simulink model "Milestone3_Code_excl4Way"  (R2023a)
settings: Solver=FixedStepDiscrete  StartTime=0.0  StopTime=50  FixedStep=0.01  RelTol=1e-3  EnableMultiTasking=on
undefined symbols (not defined in the file): DiscIntNeverNeededParam
libraries: arduinolib x14, simulink x3, hdlsllib x2, slpidlib x1, mobileRoboticsTrainingLib x1, arduinosensorlib x1
(part 2 of 2)

== stateflow chart Milestone3_Code_excl4Way/Motion Control1/Intersection Navigation1 ==
  note: Basic Description
      | Default: Curve Navigation controls the velocity and angular velocity
      |
      | When infrared sensor 1 or 4 (IR1 and IR4) detect a black line, this Intersection Navigation subsystem takes control and calls the leftTurn or rightTurn procedure respectively.
      | Intersection procedure (same for both leftTurn or rightTurn):
      | 	Increment branchCounter to keep track of the number of branches.
      | 	Move forward a small distance to align with the turn.
      | 	Rotate in the correct direction until the middle two sensors detect a line again.
      | 	Pass control to Curve Navigation to navigate the offshoot.
      | 	If the offshoot comes to an end (all sensors detect white), rotate 180 degrees and navigate back to the main path.
      | 	If the offshoot ends in a detect line (all sensors detect black), stop, send a signal to the Object Detection subsystem to measure for an object, rotate 180 degrees and navigate back to the main path.
      | 		Add branch number from branchCounter to objectMap to indicate this branch has an object.
      | 	Pass control to Curve Navigation to navigate the offshoot returning to the main path.
      | 	When the peripheral sensors detect a black line again (meaning the robot has returned to the intersection with the main branch), control is passed to Intersection Navigation.
      | 	Move forward a small distance to align with the turn.
      | 	Rotate in the correct direction until the middle two sensors detect a line again.
      | 	Pass control back to Curve Navigation to continue traversing the main path.
      |
      | If all sensors detect black whilst the robot is on the main path, the endOfMaze procedure is called.
      | endOfMaze procedure:
      | 	Stop
      | 	Use objectMap to determine how many objects were discovered.
      | 	Find the branch number of the object with the smallest distance, saved to branchWithObject.
      | 		objectCounter provides number of object with smallest distance measured.
      | 		Obtain the n'th number in objectMap to determine the branch number containing said object (where n = objectCounter)
      | 	Invert branchWithObject such that it provides the number of the branch starting from the end of the maze.
      | 	Set renavigating to HIGH.
      |
      | Renavigating Procedure:
      | 	Rotate 180 degrees to re-traverse the maze.
      | 	set branchCounter to 0.
      | 	Pass control to Curve Navigation to renavigate maze.
      | 	If intersection is detected, increment branchCounter.
      | 	If branchCounter is equal to branchWithObject at an intersection, turn into that offshoot.
      | 	Pass control to Curve Navigation to navigate offshoot.
      | 	If all sensors detect black at the "detect object line", come to a stop.
  note: Note to self:
      | Make sure all blocks with forward velocity use curve-following algorithm (never move forward blindly)
      |
      | Neaten up blocks
      |
      | Add 4way navigation
      |
      | Make back and forth smaller (will need to be adjusted for real life speed)
  state analyseIntersection
    state returnToIntersection
      entry: distance0 = distance;
      state FollowTrack
        %middle two sense black
        velocity = -0.05;
        angular_velocity = 0;
      state TurnLeft
        entry:
        velocity = 0;
        angular_velocity = -2;
      state TurnRight
        entry:
        velocity = 0;
        angular_velocity = 2;
      (default) -> analyseIntersection.returnToIntersection.FollowTrack
      analyseIntersection.returnToIntersection.TurnRight -> analyseIntersection.returnToIntersection.FollowTrack : [IR3 == 0 && IR2 == 0]
      analyseIntersection.returnToIntersection.TurnLeft -> analyseIntersection.returnToIntersection.FollowTrack : [IR3 == 0 && IR2 == 0]
      analyseIntersection.returnToIntersection.FollowTrack -> analyseIntersection.returnToIntersection.TurnRight [order 2] : [IR2 == 1]
      analyseIntersection.returnToIntersection.FollowTrack -> analyseIntersection.returnToIntersection.TurnLeft [order 1] : [IR3 == 1]
    state moveForward
      entry: distance0 = distance;
      state FollowTrack
        %middle two sense black
        velocity = 1;
        angular_velocity = 0;
      state TurnRight
        entry:
        velocity = 0;
        angular_velocity = 2;
      state TurnLeft
        entry:
        velocity = 0;
        angular_velocity = -2;
      analyseIntersection.moveForward.TurnLeft -> analyseIntersection.moveForward.FollowTrack : [IR3 == 0 && IR2 == 0]
      analyseIntersection.moveForward.FollowTrack -> analyseIntersection.moveForward.TurnLeft [order 1] : [IR3 == 1]
      analyseIntersection.moveForward.TurnRight -> analyseIntersection.moveForward.FollowTrack : [IR3 == 0 && IR2 == 0]
      analyseIntersection.moveForward.FollowTrack -> analyseIntersection.moveForward.TurnRight [order 2] : [IR2 == 1]
      (default) -> analyseIntersection.moveForward.FollowTrack
    state chooseIntersectionType
      %left turn
      %extreme left turn
      %right turn
      %extreme right turn
      %end of maze
      %4-way junction
      entry: velocity = 0;
      angular_velocity = 0;
    state commenceIntersectionControl
      entry: velocity = 0;
    (default) -> analyseIntersection.moveForward
    chooseIntersectionType -> returnToIntersection [order 2] : [(IR2 == 0 || IR3 == 0)]
    analyseIntersection.moveForward -> chooseIntersectionType : [abs(distance0 - distance) >= 0.3]
    returnToIntersection -> commenceIntersectionControl : [abs(distance0 - distance) >= 0.3]
    (junction 486) -> returnToIntersection : {finishMaze = 1;}
    chooseIntersectionType -> (junction 486) [order 3] : [IR1 + IR2 + IR3 + IR4 == 4]{fourWay = 0;}
    chooseIntersectionType -> (junction 486) [order 1] : [IR1 + IR2 + IR3 + IR4 == 0]{fourWay = 0;}
  note: if fourway doesn't work now:
      | have it pick up if another intersection is ever picked up in the slight move forward, and then limit forward movement massivly.
      | If another interesction in opposite direction was ever picked up - four way
  state endOfMaze
    %procedure to locate position of closest object once maze is completed
    entry: velocity = 0;
    angular_velocity = 0;
    num = objectMap;
    while num > 0
    len = len + 1;
    num = fix(num/10);
    end
    branchWithObject = mod(fix(objectMap/10^(len - objectCounter)), 10);
    branchWithObject = branchCounter - branchWithObject + 1
    exit:
    renavigating = 1;
  state fullRotation
    %rotate 180 degrees to renavigate maze
    entry: phi0 = phi;
    during:
    velocity = 0;
    angular_velocity = -1;
  note: if fullInter == 1:
      | if all black:
  state followMain
    state TurnRight
      entry:
      velocity = 0;
      angular_velocity = 2;
    state FollowTrack
      %middle two sense black
      velocity = 1;
      angular_velocity = 0;
    state TurnLeft
      entry:
      velocity = 0;
      angular_velocity = -2;
    (default) -> followMain.FollowTrack
    followMain.FollowTrack -> followMain.TurnLeft [order 1] : [IR3 == 1]
    followMain.TurnRight -> followMain.FollowTrack : [IR3 == 0 && IR2 == 0]
    followMain.TurnLeft -> followMain.FollowTrack : [IR3 == 0 && IR2 == 0]
    followMain.FollowTrack -> followMain.TurnRight [order 2] : [IR2 == 1]
    (junction 442) -> followMain.FollowTrack
    (junction 440) -> followMain.FollowTrack
  state Wait
  state leftTurn
    %procedure for navigating an offshoot to the right of the main path
    state Rotate
      entry:  branchCounter = branchCounter +1
      state moveForward
        entry: velocity = 1;
      state rotateOffPath
        entry:
        velocity = 0;
        angular_velocity = -1;
      state rotateOntoPath
      (default) -> leftTurn.Rotate.moveForward
      leftTurn.Rotate.moveForward -> leftTurn.Rotate.rotateOffPath : [IR1 == 1]
      leftTurn.Rotate.rotateOffPath -> (junction 365) : [IR2 == 1 && IR3 == 1]
      (junction 365) -> leftTurn.Rotate.rotateOntoPath
    state returnToMain
      state FollowTrack
        %middle two sense black
        velocity = 1;
        angular_velocity = 0;
      state TurnRight
        entry:
        velocity = 0;
        angular_velocity = 2;
      state TurnLeft1
        entry:
        velocity = 0;
        angular_velocity = -2;
      (default) -> leftTurn.returnToMain.FollowTrack
      (junction 469) -> leftTurn.returnToMain.FollowTrack
      (junction 472) -> leftTurn.returnToMain.FollowTrack
      TurnLeft1 -> (junction 469) : [IR3 == 0 && IR2 == 0]
      leftTurn.returnToMain.TurnRight -> (junction 472) : [IR3 == 0 && IR2 == 0]
      leftTurn.returnToMain.FollowTrack -> (junction 471) [order 2] : [IR2 == 1]
      leftTurn.returnToMain.FollowTrack -> (junction 470) [order 1] : [IR3 == 1]
      (junction 471) -> leftTurn.returnToMain.TurnRight
      (junction 470) -> TurnLeft1
    state leftToMain
      state moveForward
        entry: velocity = 1;
      state rotateOntoPath
      state rotateOffPath
        entry:
        velocity = 0;
        angular_velocity = 1;
      (default) -> leftTurn.leftToMain.moveForward
      leftTurn.leftToMain.moveForward -> leftTurn.leftToMain.rotateOffPath : [IR1 == 1]
      (junction 393) -> leftTurn.leftToMain.rotateOntoPath
      leftTurn.leftToMain.rotateOffPath -> (junction 393) : [IR2 == 1 && IR3 == 1]
    state navigateOffshoot
      state FollowTrack
        %middle two sense black
        velocity = 1;
        angular_velocity = 0;
      state TurnLeft
        entry:
        velocity = 0;
        angular_velocity = -2;
      state TurnRight
        entry:
        velocity = 0;
        angular_velocity = 2;
      (default) -> leftTurn.navigateOffshoot.FollowTrack
      leftTurn.navigateOffshoot.FollowTrack -> (junction 460) [order 2] : [IR2 == 1]
      (junction 460) -> leftTurn.navigateOffshoot.TurnRight
      leftTurn.navigateOffshoot.FollowTrack -> (junction 463) [order 1] : [IR3 == 1]
      (junction 463) -> leftTurn.navigateOffshoot.TurnLeft
      (junction 461) -> leftTurn.navigateOffshoot.FollowTrack : [IR3 == 0 && IR2 == 0]
      (junction 462) -> leftTurn.navigateOffshoot.FollowTrack
      leftTurn.navigateOffshoot.TurnRight -> (junction 461)
      leftTurn.navigateOffshoot.TurnLeft -> (junction 462) : [IR3 == 0 && IR2 == 0]
    state fullRotation
      %rotate 180 degrees
      entry: phi0 = phi;
      during:
      velocity = 0;
      angular_velocity = -4;
    state stopAndMeasure
      entry:
      velocity = 0;
      angular_velocity = 0;
      collectMeasurement = 1;
      exit:
      collectMeasurement = 0;
    state finalStop
      velocity = 0;
      angular_velocity = 0;
    (default) -> leftTurn.Rotate
    leftTurn.Rotate.rotateOntoPath -> leftTurn.navigateOffshoot : [IR2 == 0]
    leftTurn.returnToMain -> leftToMain : [IR1 == 0]
    leftTurn.fullRotation -> leftTurn.returnToMain : [abs(phi - phi0) > 2.793 && abs(phi - phi0) < 3.491 && IR2 == 0 && IR3 == 0]
    leftTurn.navigateOffshoot -> (junction 263) [order 2]
    (junction 263) -> (junction 264) : [IR1 + IR2 + IR3 + IR4 == 0 && renavigating == 1]
    leftTurn.navigateOffshoot -> (junction 216) [order 1] : [IR1 == 1 && IR2 == 1 && IR3 == 1 && IR4 == 1]
    (junction 216) -> leftTurn.fullRotation
    leftTurn.navigateOffshoot -> leftTurn.stopAndMeasure [order 3] : [IR1 == 0 && IR2 == 0 && IR3 == 0 && IR4 ==0]{objectMap = objectMap*10 + branchCounter;} %detect or stop line
    leftTurn.stopAndMeasure -> leftTurn.fullRotation : after(1, sec) [measurementComplete == 1]
    (junction 264) -> leftTurn.finalStop
  state rightTurn
    %procedure for navigating an offshoot to the right of the main path
    state returnToMain
      state FollowTrack
        %middle two sense black
        velocity = 1;
        angular_velocity = 0;
      state TurnLeft
        entry:
        velocity = 0;
        angular_velocity = -2;
      state TurnRight
        entry:
        velocity = 0;
        angular_velocity = 2;
      (default) -> rightTurn.returnToMain.FollowTrack
      rightTurn.returnToMain.FollowTrack -> rightTurn.returnToMain.TurnRight [order 2] : [IR2 == 1]
      rightTurn.returnToMain.TurnRight -> rightTurn.returnToMain.FollowTrack : [IR3 == 0 && IR2 == 0]
      rightTurn.returnToMain.FollowTrack -> rightTurn.returnToMain.TurnLeft [order 1] : [IR3 == 1]
      rightTurn.returnToMain.TurnLeft -> rightTurn.returnToMain.FollowTrack : [IR3 == 0 && IR2 == 0]
    state Rotate
      entry:  branchCounter = branchCounter +1
      state moveForward
        entry: velocity = 1;
      state rotateOffPath
        entry:
        velocity = 0;
        angular_velocity = 1;
      state rotateOntoPath
      (default) -> rightTurn.Rotate.moveForward
      rightTurn.Rotate.moveForward -> rightTurn.Rotate.rotateOffPath : [IR4 == 1]
      rightTurn.Rotate.rotateOffPath -> (junction 311) : [IR2 == 1 && IR3 == 1]
      (junction 311) -> rightTurn.Rotate.rotateOntoPath
    state rightToMain
      %turn right back onto the main path
      state moveForward
        entry: velocity = 1;
      state rotateOffPath
        entry:
        velocity = 0;
        angular_velocity = 1;
      state rotateOntoPath
      (default) -> rightTurn.rightToMain.moveForward
      rightTurn.rightToMain.moveForward -> rightTurn.rightToMain.rotateOffPath : [IR4 == 1]
      rightTurn.rightToMain.rotateOffPath -> (junction 357) : [IR2 == 1 && IR3 == 1]
      (junction 357) -> rightTurn.rightToMain.rotateOntoPath
    state navigateOffshoot
      state FollowTrack
        %middle two sense black
        velocity = 1;
        angular_velocity = 0;
      state TurnLeft
        entry:
        velocity = 0;
        angular_velocity = -2;
      state TurnRight1
        entry:
        velocity = 0;
        angular_velocity = 2;
      rightTurn.navigateOffshoot.FollowTrack -> (junction 448) [order 2] : [IR2 == 1]
      rightTurn.navigateOffshoot.FollowTrack -> (junction 454) [order 1] : [IR3 == 1]
      (junction 448) -> TurnRight1
      (junction 454) -> rightTurn.navigateOffshoot.TurnLeft
      (junction 450) -> rightTurn.navigateOffshoot.FollowTrack
      (default) -> rightTurn.navigateOffshoot.FollowTrack
      (junction 452) -> rightTurn.navigateOffshoot.FollowTrack
      TurnRight1 -> (junction 450) : [IR3 == 0 && IR2 == 0]
      rightTurn.navigateOffshoot.TurnLeft -> (junction 452) : [IR3 == 0 && IR2 == 0]
    state stopAndMeasure
      entry:
      velocity = 0;
      angular_velocity = 0;
      collectMeasurement = 1;
      exit:
      collectMeasurement = 0;
    state fullRotation
      %rotate 180 degrees
      entry: phi0 = phi;
      during:
      velocity = 0;
      angular_velocity = -4;
    state finalStop
      velocity = 0;
      angular_velocity = 0;
    (default) -> rightTurn.Rotate
    rightTurn.returnToMain -> rightToMain : [IR4 == 0]
    rightTurn.fullRotation -> rightTurn.returnToMain : [abs(phi - phi0) > 2.793 && abs(phi - phi0) < 3.491 && IR2 == 0 && IR3 == 0]
    rightTurn.Rotate.rotateOntoPath -> rightTurn.navigateOffshoot : [IR3 == 0]
    rightTurn.navigateOffshoot -> (junction 254) [order 1]
    (junction 254) -> (junction 256) : [IR1 + IR2 + IR3 + IR4 == 0 && renavigating == 1]
    rightTurn.navigateOffshoot -> (junction 194) [order 3] : [IR1 == 1 && IR2 == 1 && IR3 == 1 && IR4 == 1]
    (junction 194) -> rightTurn.fullRotation
    rightTurn.navigateOffshoot -> rightTurn.stopAndMeasure [order 2] : [IR1 == 0 && IR2 == 0 && IR3 == 0 && IR4 ==0]{objectMap = objectMap*10 + branchCounter;} %detect or stop line
    rightTurn.stopAndMeasure -> rightTurn.fullRotation : after(1, sec) [measurementComplete == 1]
    (junction 256) -> rightTurn.finalStop
  state renavigatingCounter
    entry:
    branchCounter = branchCounter + 1;
  commenceIntersectionControl -> endOfMaze [order 1] : [finishMaze == 1]
  endOfMaze -> fullRotation : {branchCounter = 0;}
  commenceIntersectionControl -> (junction 481) [order 3] : [IR4 == 0]
  commenceIntersectionControl -> (junction 477) [order 2] : [IR1 == 0]
  (junction 481) -> rightTurn
  (junction 477) -> leftTurn
  fullRotation -> Wait : [IR2 == 1 && IR3 == 1]
  (junction 483) -> endOfMaze
  followMain -> analyseIntersection [order 3] : [renavigating == 0 && (IR1 == 0 || IR4 == 0)]
  followMain -> analyseIntersection [order 2] : [IR1 == 0 && IR4 == 0 && renavigating == 0]{fourWay = 1;}
  (default) -> followMain
  followMain -> (junction 483) [order 1] : [IR1 + IR2 + IR3 + IR4 == 0]
  Wait -> followMain : [IR2 == 0 && IR3 == 0]
  (junction 446) -> (junction 442)
  (junction 444) -> (junction 440)
  renavigatingCounter -> followMain [order 1] : [IR1 == 1 && IR4 == 1]
  followMain -> renavigatingCounter [order 4] : [(IR1 == 0 || IR4 == 0) && renavigating == 1]
  renavigatingCounter -> leftTurn.Rotate [order 2] : [IR1 == 0 && branchCounter == branchWithObject]
  leftTurn.leftToMain.rotateOntoPath -> (junction 446) : [IR2 == 0 && IR3 == 0]
  renavigatingCounter -> rightTurn.Rotate [order 3] : [IR4 == 0 && branchCounter == branchWithObject]
  rightTurn.rightToMain.rotateOntoPath -> (junction 444) [order 2] : [IR3 == 0 && IR2 == 0]
  rightTurn.rightToMain.rotateOntoPath -> (junction 498) [order 1] : [fourWay == 1]
  (junction 498) -> leftTurn : {fourWay = 0;}
  data: len local =0; num local =0; velocity output; angular_velocity output; IR1 input; IR2 input; IR3 input; IR4 input; collectMeasurement output; phi input; phi0 local; distance input; distance0 local =0; objectCounter input; objectMap output =0; branchCounter local =0; branchWithObject local =0; renavigating local =0; measurementComplete input; finishMaze local =0; fourWay local =0
